simulink model "aerodynamic_comparison_6dof"  (R2025b)
settings: Solver=VariableStepAuto  StartTime=0.0  StopTime=10.0  RelTol=1e-3
values from neighbouring files (symbols this model uses):
  AeroData = CombinedAeroData    [initialize_sim_params_6dof.m]
  Ref_Area = RocketAeroPhysical.Reference_Area    [initialize_sim_params_6dof.m]
undefined symbols (not defined in the file or in its folder): rocket_length
libraries: aerolibconvert2 x3
settings Model: Creator=jonno  LastModifiedBy=jonno

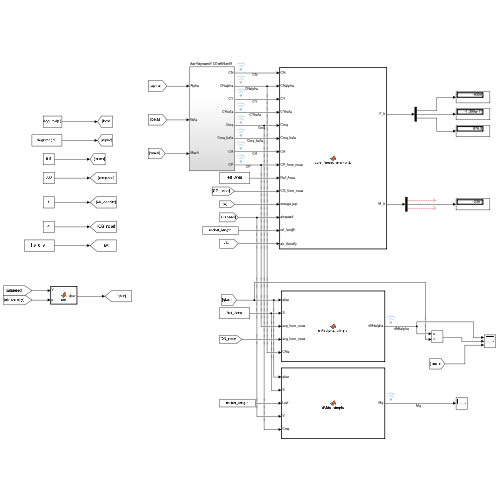
[thumbnail: Simulink's stored preview of the top-level diagram]
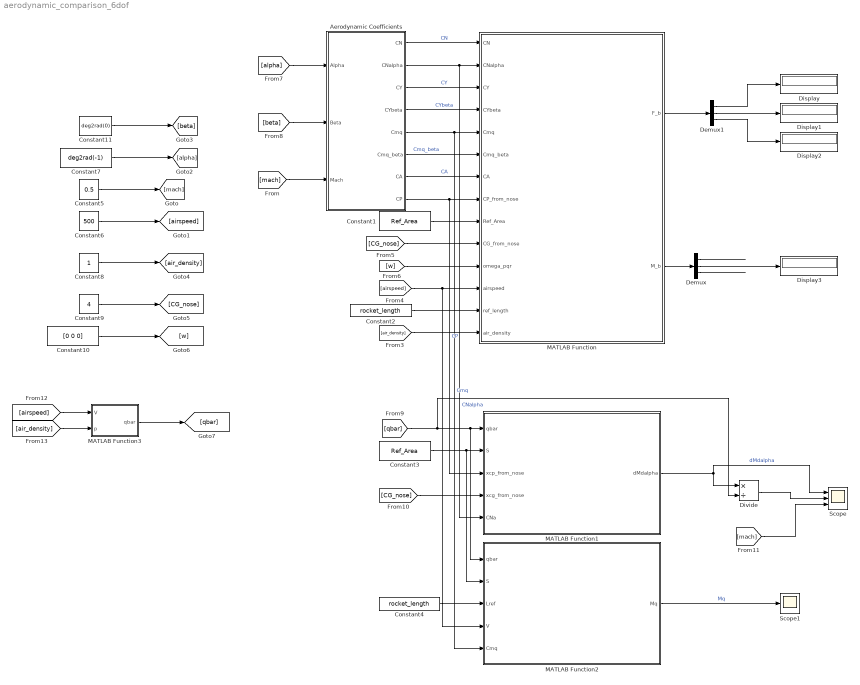
== system aerodynamic_comparison_6dof ==
  "Aerodynamic Coefficients " : Subsystem
  Constant1 : Constant  Value=Ref_Area  VectorParams1D=off
  Constant10 : Constant  Value=[0 0 0]
  Constant11 : Constant  Value=deg2rad(0)
  Constant2 : Constant  Value=rocket_length
  Constant3 : Constant  Value=Ref_Area  VectorParams1D=off
  Constant4 : Constant  Value=rocket_length
  Constant5 : Constant  Value=0.5
  Constant6 : Constant  Value=500
  Constant7 : Constant  Value=deg2rad(-1)
  Constant8 : Constant
  Constant9 : Constant  Value=4
  Demux : Demux  Outputs=3
  Demux1 : Demux  Outputs=3
  Display{,1..3} (4 alike) : Display
  Divide : Product  Inputs=*/
  MATLAB Function : MATLAB Function  TreatAsAtomicUnit=on
  MATLAB Function1 : MATLAB Function  TreatAsAtomicUnit=on
  MATLAB Function2 : MATLAB Function  TreatAsAtomicUnit=on
  MATLAB Function3 : MATLAB Function  TreatAsAtomicUnit=on
  Scope : Scope  NumInputPorts=3
      settings: ActiveDisplayYMinimum=-20269.526617708132  ActiveDisplayYMaximum=182425.7406044511  DataLoggingVariableName=ScopeData8
  Scope1 : Scope
      settings: ActiveDisplayYMinimum=-5298.2755475796475  ActiveDisplayYMaximum=588.69728306440516  DataLoggingVariableName=ScopeData9
  wires:
  "Aerodynamic Coefficients "/4(CYbeta) -> MATLAB Function/4(CYbeta)  "CYbeta"
  [CG_nose] -> MATLAB Function1/4(xcg_from_nose)
  [CG_nose] -> MATLAB Function/10(CG_from_nose)
  "Aerodynamic Coefficients "/2(CNalpha) -> MATLAB Function1/5(CNa), MATLAB Function/2(CNalpha)  "CNalpha"
  Demux/1 -> ?
  Demux/2 -> Display3/1
  [mach] -> "Aerodynamic Coefficients "/3(Mach)
  [air_density] -> MATLAB Function/14(air_density)
  MATLAB Function2/1(Mq) -> Scope1/1  "Mq"
  "Aerodynamic Coefficients "/3(CY) -> MATLAB Function/3(CY)  "CY"
  Constant3/1 -> MATLAB Function2/2(S), MATLAB Function1/2(S)
  [mach] -> Scope/3
  [alpha] -> "Aerodynamic Coefficients "/1(Alpha)
  Constant4/1 -> MATLAB Function2/3(Lref)
  MATLAB Function/1(F_b) -> Demux1/1
  MATLAB Function/2(M_b) -> Demux/1
  Divide/1 -> Scope/2
  "Aerodynamic Coefficients "/1(CN) -> MATLAB Function/1(CN)  "CN"
  MATLAB Function1/1(dMdalpha) -> Divide/1, Scope/1  "dMdalpha"
  [beta] -> "Aerodynamic Coefficients "/2(Beta)
  "Aerodynamic Coefficients "/6(Cmq_beta) -> MATLAB Function/6(Cmq_beta)  "Cmq_beta"
  [w] -> MATLAB Function/11(omega_pqr)
  "Aerodynamic Coefficients "/7(CA) -> MATLAB Function/7(CA)  "CA"
  Constant1/1 -> MATLAB Function/9(Ref_Area)
  [airspeed] -> MATLAB Function2/4(V), MATLAB Function/12(airspeed)
  Constant2/1 -> MATLAB Function/13(ref_length)
  "Aerodynamic Coefficients "/8(CP) -> MATLAB Function1/3(xcp_from_nose), MATLAB Function/8(CP_from_nose)  "CP"
  "Aerodynamic Coefficients "/5(Cmq) -> MATLAB Function2/5(Cmq), MATLAB Function/5(Cmq)  "Cmq"
  [qbar] -> Divide/2, MATLAB Function2/1(qbar), MATLAB Function1/1(qbar)
  Demux/3 -> ?
  Constant8/1 -> [air_density]
  Constant7/1 -> [alpha]
  Constant5/1 -> [mach]
  Constant6/1 -> [airspeed]
  MATLAB Function3/1(qbar) -> [qbar]
  Constant10/1 -> [w]
  [air_density] -> MATLAB Function3/2(p)
  Constant9/1 -> [CG_nose]
  [airspeed] -> MATLAB Function3/1(V)
  Constant11/1 -> [beta]
  Demux1/1 -> Display/1
  Demux1/2 -> Display1/1
  Demux1/3 -> Display2/1

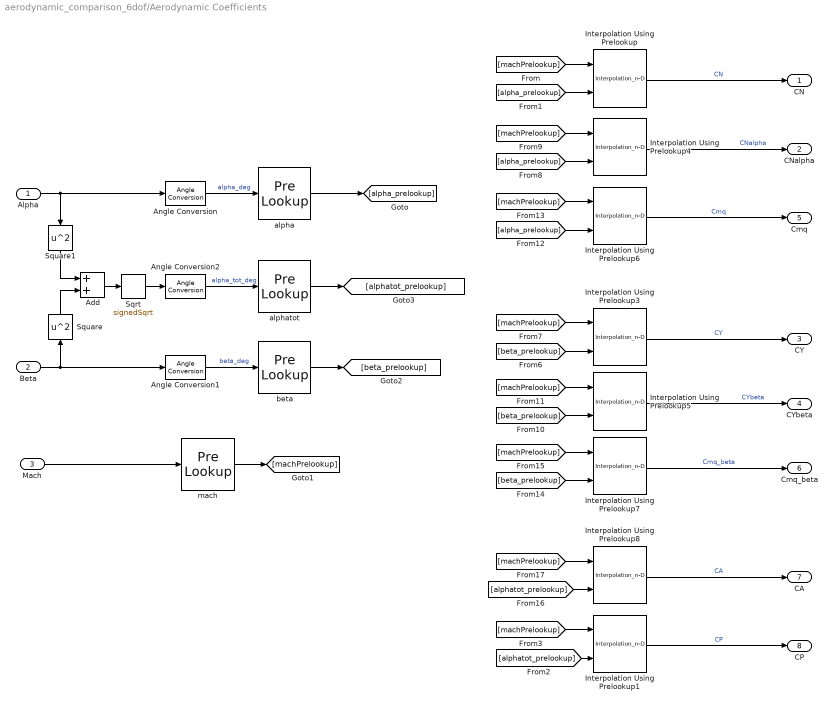
== system aerodynamic_comparison_6dof/Aerodynamic Coefficients  ==
  Alpha : Inport
  Beta : Inport  Port=2
  Mach : Inport  Port=3
  Add : Sum
  Angle Conversion : aerolibconvert2/Angle Conversion  IU=rad  OU=deg
  Angle Conversion1 : aerolibconvert2/Angle Conversion  IU=rad  OU=deg
  Angle Conversion2 : aerolibconvert2/Angle Conversion  IU=rad  OU=deg
  Interpolation Using Prelookup : Interpolation_n-D  Table=AeroData.Tables.CN  RequireIndexFractionAsBus=on  InternalRulePriority=Speed
      settings: InputPortMap=u0,u1
  Interpolation Using Prelookup1 : Interpolation_n-D  Table=AeroData.Tables.CP  RequireIndexFractionAsBus=on  InternalRulePriority=Speed
      settings: InputPortMap=u0,u1
  Interpolation Using Prelookup3 : Interpolation_n-D  Table=AeroData.Tables.CY  RequireIndexFractionAsBus=on  InternalRulePriority=Speed
      settings: InputPortMap=u0,u1
  Interpolation Using Prelookup4 : Interpolation_n-D  Table=AeroData.Tables.CNalpha  RequireIndexFractionAsBus=on  InternalRulePriority=Speed
      settings: InputPortMap=u0,u1
  Interpolation Using Prelookup5 : Interpolation_n-D  Table=AeroData.Tables.CYbeta  RequireIndexFractionAsBus=on  InternalRulePriority=Speed
      settings: InputPortMap=u0,u1
  Interpolation Using Prelookup6 : Interpolation_n-D  Table=AeroData.Tables.Cmq  RequireIndexFractionAsBus=on  InternalRulePriority=Speed
      settings: InputPortMap=u0,u1
  Interpolation Using Prelookup7 : Interpolation_n-D  Table=AeroData.Tables.Cmq_beta  RequireIndexFractionAsBus=on  InternalRulePriority=Speed
      settings: InputPortMap=u0,u1
  Interpolation Using Prelookup8 : Interpolation_n-D  Table=AeroData.Tables.CA  RequireIndexFractionAsBus=on  InternalRulePriority=Speed
      settings: InputPortMap=u0,u1
  Sqrt : Sqrt  Operator=signedSqrt
  Square : Math  Operator=square
  Square1 : Math  Operator=square
  alpha : PreLookup  BreakpointsData=AeroData.Breakpoints.Alpha  OutputSelection=Index and fraction as bus  IndexSearchMethod=Evenly spaced points  UseLastBreakpoint=on
  alphatot : PreLookup  BreakpointsData=AeroData.Breakpoints.AlphaTot  OutputSelection=Index and fraction as bus  IndexSearchMethod=Evenly spaced points  UseLastBreakpoint=on
  beta : PreLookup  BreakpointsData=AeroData.Breakpoints.Beta  OutputSelection=Index and fraction as bus  IndexSearchMethod=Evenly spaced points  UseLastBreakpoint=on
  mach : PreLookup  BreakpointsData=AeroData.Breakpoints.Mach  OutputSelection=Index and fraction as bus  IndexSearchMethod=Evenly spaced points  ExtrapMethod=Linear
  CN : Outport
  CNalpha : Outport  Port=2
  CY : Outport  Port=3
  CYbeta : Outport  Port=4
  Cmq : Outport  Port=5
  Cmq_beta : Outport  Port=6
  CA : Outport  Port=7
  CP : Outport  Port=8
  wires:
  Interpolation Using Prelookup/1 -> CN/1  "CN"
  alpha/1 -> [alpha_prelookup]
  mach/1 -> [machPrelookup]
  [machPrelookup] -> Interpolation Using Prelookup/1
  [alpha_prelookup] -> Interpolation Using Prelookup/2
  Angle Conversion/1 -> alpha/1  "alpha_deg"
  Mach/1 -> mach/1
  Alpha/1 -> Square1/1, Angle Conversion/1
  Beta/1 -> Square/1, Angle Conversion1/1
  Angle Conversion1/1 -> beta/1  "beta_deg"
  beta/1 -> [beta_prelookup]
  Add/1 -> Sqrt/1
  Square1/1 -> Add/1
  Square/1 -> Add/2
  alphatot/1 -> [alphatot_prelookup]
  Angle Conversion2/1 -> alphatot/1  "alpha_tot_deg"
  Sqrt/1 -> Angle Conversion2/1
  [alpha_prelookup] -> Interpolation Using Prelookup4/2
  [machPrelookup] -> Interpolation Using Prelookup4/1
  Interpolation Using Prelookup4/1 -> CNalpha/1  "CNalpha"
  [machPrelookup] -> Interpolation Using Prelookup3/1
  [beta_prelookup] -> Interpolation Using Prelookup3/2
  Interpolation Using Prelookup3/1 -> CY/1  "CY"
  [machPrelookup] -> Interpolation Using Prelookup5/1
  Interpolation Using Prelookup5/1 -> CYbeta/1  "CYbeta"
  [beta_prelookup] -> Interpolation Using Prelookup5/2
  [machPrelookup] -> Interpolation Using Prelookup6/1
  [alpha_prelookup] -> Interpolation Using Prelookup6/2
  Interpolation Using Prelookup6/1 -> Cmq/1  "Cmq"
  [machPrelookup] -> Interpolation Using Prelookup7/1
  Interpolation Using Prelookup7/1 -> Cmq_beta/1  "Cmq_beta"
  [beta_prelookup] -> Interpolation Using Prelookup7/2
  [machPrelookup] -> Interpolation Using Prelookup8/1
  Interpolation Using Prelookup8/1 -> CA/1  "CA"
  [alphatot_prelookup] -> Interpolation Using Prelookup8/2
  Interpolation Using Prelookup1/1 -> CP/1  "CP"
  [alphatot_prelookup] -> Interpolation Using Prelookup1/2
  [machPrelookup] -> Interpolation Using Prelookup1/1

== matlab function aerodynamic_comparison_6dof/MATLAB Function3 ==
  data: V input; qbar output; p input
function qbar = fcn(V, p)



qbar = (1/2)*V^2 * p;

== matlab function aerodynamic_comparison_6dof/MATLAB Function ==
  data: CN input; F_b output; CNalpha input; CY input; CYbeta input; Cmq input; Cmq_beta input; CA input; CP_from_nose input; Ref_Area input; CG_from_nose input; omega_pqr input; airspeed input; ref_length input; air_density input; M_b output
function [F_b, M_b] = aero_forces_moments( ...
    CN, CNalpha, CY, CYbeta, Cmq, Cmq_beta, CA, CP_from_nose, ...
    Ref_Area, CG_from_nose, omega_pqr, airspeed, ref_length, air_density)
% Aero forces and moments (body axes), with beta convention:
%   Positive beta = wind from the right
% Inputs:
%   CN, CY, CA             : force coefficients
%   CNalpha, CYbeta        : slopes (reserved)
%   Cmq, Cmq_beta          : damping (pitch/yaw), lumped
%   CP_from_nose, CG_from_nose : [m]
%   Ref_Area               : [m^2]
%   ref_length             : [m]
%   omega_pqr              : [rad/s] [p; q; r]
%   airspeed               : [m/s]
%   air_density            : [kg/m^3]
% Outputs:
%   F_b = [Fx; Fy; Fz], M_b = [Mx; My; Mz]



% --- Precompute
S  = Ref_Area;
d  = ref_length;
V  = max(airspeed, 1e-6);
q_dyn = 0.5 * air_density * V * V;
Lcp = CP_from_nose - CG_from_nose;

% Body rates
p = omega_pqr(1);
q = omega_pqr(2);
r = omega_pqr(3);

% --- Adjust lateral force for beta sign convention (positive beta = wind from right)
CY_eff = -CY;

% --- Forces (x forward, y right, z down)
Fx = - q_dyn * S * CA;
Fy =   q_dyn * S * CY_eff;
Fz = - q_dyn * S * CN;

% --- Static moments from CP lever arm
M_stat_x = 0.0;
M_stat_y = - q_dyn * S * CN     * Lcp;
M_stat_z = - q_dyn * S * CY_eff * Lcp;

% --- Rate damping with d/(2V) (Cmq and Cmq_beta are negative for damping, keep as-is)
scale = d / (2.0 * V);
M_damp_y = q_dyn * S * d * ( scale * Cmq      * q );
M_damp_z = q_dyn * S * d * ( scale * Cmq_beta * r );

% --- Totals
Mx = M_stat_x;
My = M_stat_y + M_damp_y;
Mz = M_stat_z + M_damp_z;

F_b = [Fx; Fy; Fz];
M_b = [Mx; My; Mz];
end

== matlab function aerodynamic_comparison_6dof/MATLAB Function1 ==
  data: qbar input; S input; xcp_from_nose input; xcg_from_nose input; CNa input; dMdalpha output
function dMdalpha = dMdalpha_simple(qbar, S, xcp_from_nose, xcg_from_nose, CNa)
% --- Aero pitching-moment derivative about CG [N*m/rad]
% Inputs (SI): qbar [N/m^2], S [m^2], xcp_from_nose [m], xcg_from_nose [m], CNa [1/rad]
% Coordinates: x measured from nose toward tail

% lever arm CP minus CG
lever = xcg_from_nose - xcp_from_nose;

% small-angle aero moment derivative
dMdalpha = qbar * S * lever * CNa;
end

== matlab function aerodynamic_comparison_6dof/MATLAB Function2 ==
  data: qbar input; S input; Lref input; V input; Cmq input; Mq output
function Mq = dMdq_simple(qbar, S, Lref, V, Cmq)
% --- Aero pitch-rate damping derivative M_q [N*m/(rad/s)]
% Inputs (SI):
%   qbar : dynamic pressure [N/m^2]
%   S    : reference area [m^2]
%   Lref : reference length (e.g., diameter/chord) [m]
%   V    : true airspeed [m/s]
%   Cmq  : pitching-moment coefficient derivative wrt pitch rate (dimensionless)
%
% Output:
%   Mq   : dM/dq [N*m/(rad/s)]

Mq = qbar * S * (Lref^2 / (2*max(V, eps))) * Cmq;
end
